simulink model "quarterCar_LQR"  (R2026a)
settings: Solver=VariableStepAuto
undefined symbols (not defined in the file): K

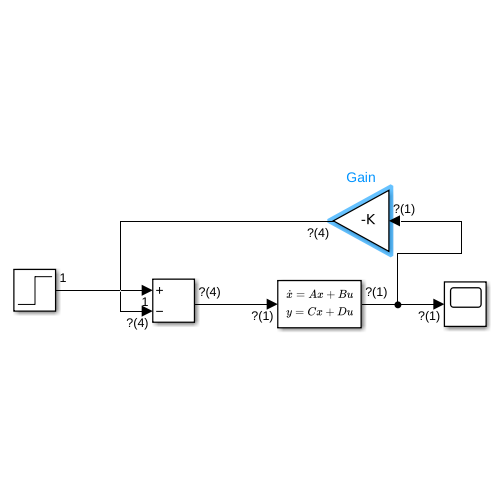
[thumbnail: Simulink's stored preview of the top-level diagram]
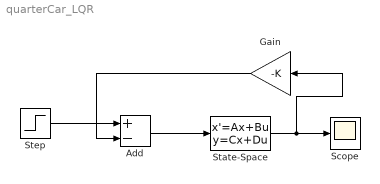
== system quarterCar_LQR ==
  Add : Sum  Inputs=+-
  Gain : Gain  Gain=-K
  Scope : Scope
      settings: ActiveDisplayYMinimum=-1  ActiveDisplayYMaximum=1
  State-Space : StateSpace  InitialCondition=0
  Step : Step  SampleTime=0
  wires:
  Step/1 -> Add/1
  Add/1 -> State-Space/1
  State-Space/1 -> Gain/1, Scope/1
  Gain/1 -> Add/2
